simulink model "SIL_OlfatiSaber"  (R2021b)
settings: Solver=FixedStepDiscrete  StartTime=0  StopTime=T  FixedStep=0.01  RelTol=1e-3  EnableMultiTasking=on
model workspace (MAT data in the model file):
  SL_ROS_VariableLengthArrays_MaxSizes : object (value not decoded)
values from neighbouring files (symbols this model uses):
  airspeed_ref = 42    [start_swarm.m]
  altitude_ref = 300    [start_swarm.m]
  N_Waypoints = size(Waypoints,1)    [start_swarm.m]
  radius_waypoint = 200    [start_swarm.m]
  Waypoints = [1200 -1000 ... (first row only)    [start_swarm.m]
undefined symbols (not defined in the file or in its folder): DiscIntNeverNeededParam, Elevators, p_swarm, Propeller, RightAileron, RightFlap, Rudder
libraries: robotlib x36, slpidlib x15, eeGeneralControl x5, simulink x5
(part 3 of 5)

== system SIL_OlfatiSaber/UAV 5/Low-level/Guidance Algorithm ==
  yaw : Inport
  x : Inport  Port=2
  y : Inport  Port=3
  x ref : Inport  Port=4
  y ref : Inport  Port=5
  Atan2 : Trigonometry  Operator=atan2
  Constant : Constant
  Constant1 : Constant  Value=0
  Constant2 : Constant  Value=1.2
  Constant3 : Constant  Value=10
  Discrete PID : slpidlib/PID Controller  Controller=PID  Form=Parallel  TimeDomain=Discrete-time  UseExternalTs=off  SampleTime=-1  IntegratorMethod=Forward Euler  FilterMethod=Forward Euler  ControllerParametersSource=external  P=1  I=1  D=0  UseFilter=on  N=100  TunerSelectOption=Transfer Function Based (PID Tuner App)  InitialConditionSource=internal  InitialConditionForIntegrator=0  InitialConditionForFilter=0  DifferentiatorICPrevScaledInput=0  ExternalReset=none  TrackingMode=off  Kt=1  LimitOutput=off  SatLimitsSource=internal  UpperSaturationLimit=inf  LowerSaturationLimit=-inf  LinearizeAsGain=on  AntiWindupMode=none  Kb=1  POutMin=[]  POutMax=[]  IOutMin=[]  IOutMax=[]  DOutMin=[]  DOutMax=[]  NOutMin=[]  NOutMax=[]  SumOutMin=[]  SumOutMax=[]  SaturationOutMin=[]  SaturationOutMax=[]  PParamMin=[]  PParamMax=[]  IParamMin=[]  IParamMax=[]  DParamMin=[]  DParamMax=[]  NParamMin=[]  NParamMax=[]  KbParamMin=[]  KbParamMax=[]  KtParamMin=[]  KtParamMax=[]  KbOutMin=[]  KbOutMax=[]  KtOutMin=[]  KtOutMax=[]  IntegratorOutMin=[]  IntegratorOutMax=[]  FilterOutMin=[]  FilterOutMax=[]  SumI1OutMin=[]  SumI1OutMax=[]  SumI2OutMin=[]  SumI2OutMax=[]  SumI3OutMin=[]  SumI3OutMax=[]  SumI4OutMin=[]  SumI4OutMax=[]  SumDOutMin=[]  SumDOutMax=[]  DifferentiatorOutMin=[]  DifferentiatorOutMax=[]  FilterDiffOutCoefMin=[]  FilterDiffOutCoefMax=[]  ReciprocalOutMin=[]  ReciprocalOutMax=[]  SumDenOutMin=[]  SumDenOutMax=[]  SumNumOutMin=[]  SumNumOutMax=[]  DivideOutMin=[]  DivideOutMax=[]  UdiffTsProdOutMin=[]  UdiffTsProdOutMax=[]  NTsProdOutMin=[]  NTsProdOutMax=[]  UintegralTsProdOutMin=[]  UintegralTsProdOutMax=[]  UngainTsProdOutMin=[]  UngainTsProdOutMax=[]  IntegratorContinuousStateAttributes=''  IntegratorStateMustResolveToSignalObject=off  IntegratorRTWStateStorageClass=Auto  FilterContinuousStateAttributes=''  FilterStateMustResolveToSignalObject=off  FilterRTWStateStorageClass=Auto  ParallelPVariant=ExternalParameters  IdealPVariant=Disabled  IVariant=ExternalParameters  DVariant=ExternalParameters  IntegratorVariant=Discrete  SatVariant=Disabled  AWVariant=Passthrough  PCopyVariant=Disabled  TRVariant=Disabled  FdbkBlocksVariant=Forward  IdealPFdbkVariant=Disabled  SatFdbkVariant=Disabled  DerivativeFilterVariant=ForwardEulerFilter  NVariant=ExternalParameters  NCopyVariant=Disabled  FilterICVariant=InternalICsFilter  IntegratorICVariant=InternalICs  ExternalResetVariant=Disabled  TRSumVariant=Passthrough  SumFdbkVariant=Disabled  SumVariant=Sum_PID  TsampFilterVariant=InternalTs  TsampNgainVariant=Passthrough  TsampIntegralVariant=Passthrough  ExternalSaturationOutDataTypeStr=Inherit: Same as second input
  Gain : Gain  Gain=1.67
  Gain1 : Gain  Gain=-1
  Mux1 : Mux  Inputs=2
  Mux2 : Mux  Inputs=2
  Mux3 : Mux  Inputs=2
  Saturation : Saturate  UpperLimit=0.226893  LowerLimit=-0.226893
  Sum2 : Sum  Inputs=|+-
  Sum3 : Sum  Inputs=|+-
  Sum4 : Sum  Inputs=|+-
  roll_ref : Outport
  yaw_error : Outport  Port=2
  positions : Outport  Port=3
  wires:
  Mux1/1 -> Mux3/1
  Mux2/1 -> Mux3/2
  Saturation/1 -> Gain1/1
  Sum3/1 -> Atan2/1
  y/1 -> Sum3/2, Mux2/2
  y ref/1 -> Mux2/1, Sum3/1
  x ref/1 -> Mux1/1, Sum2/1
  x/1 -> Sum2/2, Mux1/2
  Sum2/1 -> Atan2/2
  Atan2/1 -> Sum4/1
  yaw/1 -> Sum4/2
  Mux3/1 -> positions/1
  Discrete PID/1 -> Saturation/1
  Sum4/1 -> yaw_error/1, Gain/1
  Gain1/1 -> roll_ref/1
  Constant/1 -> Discrete PID/2
  Constant1/1 -> Discrete PID/3
  Constant2/1 -> Discrete PID/4
  Constant3/1 -> Discrete PID/5
  Gain/1 -> Discrete PID/1

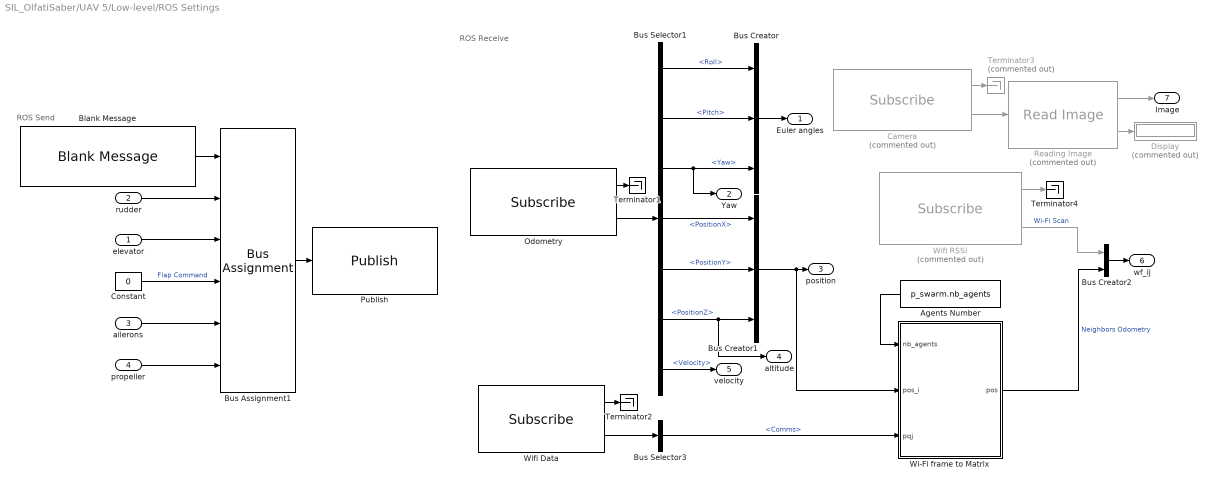
== system SIL_OlfatiSaber/UAV 5/Low-level/ROS Settings ==
  note: ROS Receive
  note: ROS Send
  elevator : Inport
  rudder : Inport  Port=2
  ailerons : Inport  Port=3
  propeller : Inport  Port=4
  Agents Number : Constant  Value=p_swarm.nb_agents
  Blank Message : robotlib/Blank Message  messageClass=Message  entityType=cosmus_messages/Control_Surfaces  messageType=cosmus_messages/Control_Surfaces  SampleTime=-1  legacyBusStruct=off
  Bus Assignment1 : BusAssignment  AssignedSignals=Rudder,Elevators,RightFlap,RightAileron,Propeller
  Bus Creator : BusCreator  Inputs=3
  Bus Creator1 : BusCreator  Inputs=3
  Bus Creator2 : BusCreator  Inputs=2
  Bus Selector1 : BusSelector  OutputSignals=Roll,Pitch,Yaw,PositionX,PositionY,PositionZ,Velocity
  Bus Selector3 : BusSelector  OutputSignals=Comms
  Camera : robotlib/Subscribe  Commented=on  topicSource=Select from ROS network  topic=/uav1/camera/image_raw  messageType=sensor_msgs/Image  SampleTime=-1  legacyBusStruct=off  messageQueueLength=1
  Constant : Constant  Value=0
  Display : Display  Commented=on
  Odometry : robotlib/Subscribe  topicSource=Select from ROS network  topic=/uav5/ground_truth/Odometry  messageType=cosmus_communication/Odom  SampleTime=-1  legacyBusStruct=off  messageQueueLength=1
  Publish : robotlib/Publish  topicSource=Select from ROS network  topic=/uav5/command  messageType=cosmus_messages/Control_Surfaces  legacyBusStruct=off  messageQueueLength=1
  Reading Image : robotlib/Read Image  Commented=on  MaximumImageSize=[240, 360]  ImageEncoding=rgb8  ShowAlphaOutput=off  ShowErrorCodeOutput=on  VariableSizeOutputs=off
      settings: SourceProductBaseCode=RR
  Terminator1 : Terminator
  Terminator2 : Terminator
  Terminator3 : Terminator  Commented=on
  Terminator4 : Terminator
  Wi-Fi frame to Matrix : MATLAB Function  TreatAsAtomicUnit=on
  Wifi Data : robotlib/Subscribe  topicSource=Select from ROS network  topic=/uav5/wifi_receiver/data  messageType=cosmus_messages/NetworkComm  SampleTime=-1  legacyBusStruct=off  messageQueueLength=1
  Wifi RSSI : robotlib/Subscribe  Commented=on  topicSource=Select from ROS network  topic=/uav1/wifi_receiver/wifi_scan  messageType=cosmus_messages/WifiSignals  SampleTime=-1  legacyBusStruct=off  messageQueueLength=1
  Euler angles : Outport
  Yaw : Outport  Port=2
  position : Outport  Port=3
  altitude : Outport  Port=4
  velocity : Outport  Port=5
  wf_ij : Outport  Port=6
  Image : Outport  Port=7
  wires:
  Odometry/1 -> Terminator1/1
  Blank Message/1 -> Bus Assignment1/1
  Bus Selector1/3 -> Bus Creator/3, Yaw/1  "<Yaw>"
  Bus Creator/1 -> Euler angles/1
  Bus Selector1/1 -> Bus Creator/1  "<Roll>"
  Bus Selector1/2 -> Bus Creator/2  "<Pitch>"
  Constant/1 -> Bus Assignment1/4  "Flap Command"
  Bus Assignment1/1 -> Publish/1
  Odometry/2 -> Bus Selector1/1
  Bus Selector1/4 -> Bus Creator1/1  "<PositionX>"
  Bus Selector1/5 -> Bus Creator1/2  "<PositionY>"
  Bus Selector1/6 -> Bus Creator1/3, altitude/1  "<PositionZ>"
  propeller/1 -> Bus Assignment1/6
  ailerons/1 -> Bus Assignment1/5
  elevator/1 -> Bus Assignment1/3
  Bus Selector1/7 -> velocity/1  "<Velocity>"
  rudder/1 -> Bus Assignment1/2
  Wifi Data/1 -> Terminator2/1
  Wifi Data/2 -> Bus Selector3/1
  Bus Selector3/1 -> Wi-Fi frame to Matrix/3(pqj)  "<Comms>"
  Agents Number/1 -> Wi-Fi frame to Matrix/1(nb_agents)
  Bus Creator1/1 -> position/1, Wi-Fi frame to Matrix/2(pos_i)
  Wi-Fi frame to Matrix/1(pos) -> Bus Creator2/2  "Neighbors Odometry"
  Camera/2 -> Reading Image/1
  Reading Image/1 -> Image/1
  Reading Image/2 -> Display/1
  Camera/1 -> Terminator3/1
  Wifi RSSI/1 -> Terminator4/1
  Wifi RSSI/2 -> Bus Creator2/1  "Wi-Fi Scan"
  Bus Creator2/1 -> wf_ij/1

== system SIL_OlfatiSaber/UAV 5/Low-level/Vision ==
  Image : Inport
  Video Viewer : VideoViewer  Commented=on  FigPos=[505 744 418 304]
  wires:
  Image/1 -> Video Viewer/1

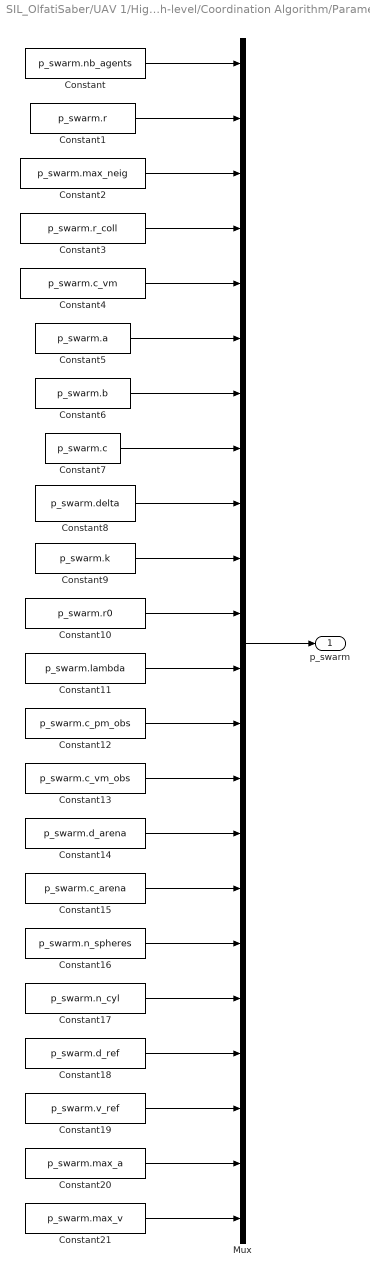
== system SIL_OlfatiSaber/UAV 1/High-level/Coordination Algorithm/Parameters ==
  Constant : Constant  Value=p_swarm.nb_agents
  Constant1 : Constant  Value=p_swarm.r
  Constant10 : Constant  Value=p_swarm.r0
  Constant11 : Constant  Value=p_swarm.lambda
  Constant12 : Constant  Value=p_swarm.c_pm_obs
  Constant13 : Constant  Value=p_swarm.c_vm_obs
  Constant14 : Constant  Value=p_swarm.d_arena
  Constant15 : Constant  Value=p_swarm.c_arena
  Constant16 : Constant  Value=p_swarm.n_spheres
  Constant17 : Constant  Value=p_swarm.n_cyl
  Constant18 : Constant  Value=p_swarm.d_ref
  Constant19 : Constant  Value=p_swarm.v_ref
  Constant2 : Constant  Value=p_swarm.max_neig
  Constant20 : Constant  Value=p_swarm.max_a
  Constant21 : Constant  Value=p_swarm.max_v
  Constant3 : Constant  Value=p_swarm.r_coll
  Constant4 : Constant  Value=p_swarm.c_vm
  Constant5 : Constant  Value=p_swarm.a
  Constant6 : Constant  Value=p_swarm.b
  Constant7 : Constant  Value=p_swarm.c
  Constant8 : Constant  Value=p_swarm.delta
  Constant9 : Constant  Value=p_swarm.k
  Mux : Mux  Inputs=22
  p_swarm : Outport
  wires:
  Mux/1 -> p_swarm/1
  Constant21/1 -> Mux/22
  Constant20/1 -> Mux/21
  Constant19/1 -> Mux/20
  Constant18/1 -> Mux/19
  Constant17/1 -> Mux/18
  Constant16/1 -> Mux/17
  Constant15/1 -> Mux/16
  Constant14/1 -> Mux/15
  Constant13/1 -> Mux/14
  Constant12/1 -> Mux/13
  Constant11/1 -> Mux/12
  Constant10/1 -> Mux/11
  Constant9/1 -> Mux/10
  Constant8/1 -> Mux/9
  Constant7/1 -> Mux/8
  Constant6/1 -> Mux/7
  Constant5/1 -> Mux/6
  Constant4/1 -> Mux/5
  Constant3/1 -> Mux/4
  Constant2/1 -> Mux/3
  Constant1/1 -> Mux/2
  Constant/1 -> Mux/1

== system SIL_OlfatiSaber/UAV 1/Low-level/Autopilot/Altitude Control ==
  Altitude Ref : Inport
  Altitude : Inport  Port=2
  Constant : Constant
  Constant1 : Constant  Value=0.00
  Constant2 : Constant  Value=0.0162
  Constant3 : Constant  Value=10
  Discrete PID : slpidlib/PID Controller  Controller=PID  Form=Parallel  TimeDomain=Discrete-time  UseExternalTs=off  SampleTime=-1  IntegratorMethod=Forward Euler  FilterMethod=Forward Euler  ControllerParametersSource=external  P=1  I=1  D=0  UseFilter=on  N=100  TunerSelectOption=Transfer Function Based (PID Tuner App)  InitialConditionSource=internal  InitialConditionForIntegrator=0  InitialConditionForFilter=0  DifferentiatorICPrevScaledInput=0  ExternalReset=none  TrackingMode=off  Kt=1  LimitOutput=off  SatLimitsSource=internal  UpperSaturationLimit=inf  LowerSaturationLimit=-inf  LinearizeAsGain=on  AntiWindupMode=none  Kb=1  POutMin=[]  POutMax=[]  IOutMin=[]  IOutMax=[]  DOutMin=[]  DOutMax=[]  NOutMin=[]  NOutMax=[]  SumOutMin=[]  SumOutMax=[]  SaturationOutMin=[]  SaturationOutMax=[]  PParamMin=[]  PParamMax=[]  IParamMin=[]  IParamMax=[]  DParamMin=[]  DParamMax=[]  NParamMin=[]  NParamMax=[]  KbParamMin=[]  KbParamMax=[]  KtParamMin=[]  KtParamMax=[]  KbOutMin=[]  KbOutMax=[]  KtOutMin=[]  KtOutMax=[]  IntegratorOutMin=[]  IntegratorOutMax=[]  FilterOutMin=[]  FilterOutMax=[]  SumI1OutMin=[]  SumI1OutMax=[]  SumI2OutMin=[]  SumI2OutMax=[]  SumI3OutMin=[]  SumI3OutMax=[]  SumI4OutMin=[]  SumI4OutMax=[]  SumDOutMin=[]  SumDOutMax=[]  DifferentiatorOutMin=[]  DifferentiatorOutMax=[]  FilterDiffOutCoefMin=[]  FilterDiffOutCoefMax=[]  ReciprocalOutMin=[]  ReciprocalOutMax=[]  SumDenOutMin=[]  SumDenOutMax=[]  SumNumOutMin=[]  SumNumOutMax=[]  DivideOutMin=[]  DivideOutMax=[]  UdiffTsProdOutMin=[]  UdiffTsProdOutMax=[]  NTsProdOutMin=[]  NTsProdOutMax=[]  UintegralTsProdOutMin=[]  UintegralTsProdOutMax=[]  UngainTsProdOutMin=[]  UngainTsProdOutMax=[]  IntegratorContinuousStateAttributes=''  IntegratorStateMustResolveToSignalObject=off  IntegratorRTWStateStorageClass=Auto  FilterContinuousStateAttributes=''  FilterStateMustResolveToSignalObject=off  FilterRTWStateStorageClass=Auto  ParallelPVariant=ExternalParameters  IdealPVariant=Disabled  IVariant=ExternalParameters  DVariant=ExternalParameters  IntegratorVariant=Discrete  SatVariant=Disabled  AWVariant=Passthrough  PCopyVariant=Disabled  TRVariant=Disabled  FdbkBlocksVariant=Forward  IdealPFdbkVariant=Disabled  SatFdbkVariant=Disabled  DerivativeFilterVariant=ForwardEulerFilter  NVariant=ExternalParameters  NCopyVariant=Disabled  FilterICVariant=InternalICsFilter  IntegratorICVariant=InternalICs  ExternalResetVariant=Disabled  TRSumVariant=Passthrough  SumFdbkVariant=Disabled  SumVariant=Sum_PID  TsampFilterVariant=InternalTs  TsampNgainVariant=Passthrough  TsampIntegralVariant=Passthrough  ExternalSaturationOutDataTypeStr=Inherit: Same as second input
  Gain : Gain  Gain=0.1
  Saturation : Saturate  UpperLimit=0.78  LowerLimit=-0.78
  Sum : Sum  Inputs=|+-
  Pitch_ref : Outport
  altitude_error : Outport  Port=2
  wires:
  Saturation/1 -> Pitch_ref/1
  Altitude Ref/1 -> Sum/1
  Altitude/1 -> Sum/2
  Sum/1 -> altitude_error/1, Gain/1
  Constant/1 -> Discrete PID/2
  Constant1/1 -> Discrete PID/3
  Constant2/1 -> Discrete PID/4
  Constant3/1 -> Discrete PID/5
  Discrete PID/1 -> Saturation/1
  Gain/1 -> Discrete PID/1

== system SIL_OlfatiSaber/UAV 1/Low-level/Autopilot/Attitude Control ==
  Pitch Ref : Inport
  Roll_ref : Inport  Port=2
  Euler angles : Inport  Port=3
  Bus Selector1 : BusSelector  OutputSignals=Pitch,Yaw,Roll
  Sum1 : Sum  Inputs=|+-
  Sum3 : Sum  Inputs=+-|
  Terminator : Terminator
  pitch_error : Outport
  roll_error : Outport  Port=2
  wires:
  Euler angles/1 -> Bus Selector1/1
  Sum1/1 -> roll_error/1
  Sum3/1 -> pitch_error/1
  Roll_ref/1 -> Sum1/1
  Bus Selector1/1 -> Sum3/2  "<Pitch>"
  Pitch Ref/1 -> Sum3/1
  Bus Selector1/3 -> Sum1/2  "<Roll>"
  Bus Selector1/2 -> Terminator/1  "<Yaw>"

== system SIL_OlfatiSaber/UAV 1/Low-level/Autopilot/Takeoff ==
  Elevator Command : Inport
  Ailerons Command : Inport  Port=2
  Propeller Command : Inport  Port=3
  Altitude : Inport  Port=4
  Constant1 : Constant  Value=0.0436332
  Constant2 : Constant  Value=0.017
  Constant3 : Constant  Value=0.8
  Constant4 : Constant  Value=0
  Constant5 : Constant  Value=-0.035
  GreaterThanOrEqual : RelationalOperator  OutDataTypeStr=boolean  RndMeth=Simplest
  Switch{1..4} (4 alike) : Switch  Criteria=u2 ~= 0
  altitude takeoff : Constant  Value=5
  profundor : Outport
  aileron : Outport  Port=2
  throtlle : Outport  Port=3
  rudder : Outport  Port=4
  wires:
  Elevator Command/1 -> Switch3/1
  Switch3/1 -> profundor/1
  Ailerons Command/1 -> Switch1/1
  Switch1/1 -> aileron/1
  Switch2/1 -> throtlle/1
  Propeller Command/1 -> Switch2/1
  Constant1/1 -> Switch3/3
  Constant2/1 -> Switch1/3
  Constant3/1 -> Switch2/3
  altitude takeoff/1 -> GreaterThanOrEqual/2
  Altitude/1 -> GreaterThanOrEqual/1
  GreaterThanOrEqual/1 -> Switch4/2, Switch3/2, Switch1/2, Switch2/2
  Constant4/1 -> Switch4/1
  Constant5/1 -> Switch4/3
  Switch4/1 -> rudder/1

== system SIL_OlfatiSaber/UAV 1/Low-level/Autopilot/Velocity Control ==
  Velocity Ref : Inport
  Velocity : Inport  Port=2
  Constant : Constant
  Constant1 : Constant  Value=0.00
  Constant2 : Constant  Value=0.009
  Constant3 : Constant  Value=10
  Discrete PID : slpidlib/PID Controller  Controller=PID  Form=Parallel  TimeDomain=Discrete-time  UseExternalTs=off  SampleTime=-1  IntegratorMethod=Forward Euler  FilterMethod=Forward Euler  ControllerParametersSource=external  P=1  I=1  D=0  UseFilter=on  N=100  TunerSelectOption=Transfer Function Based (PID Tuner App)  InitialConditionSource=internal  InitialConditionForIntegrator=0  InitialConditionForFilter=0  DifferentiatorICPrevScaledInput=0  ExternalReset=none  TrackingMode=off  Kt=1  LimitOutput=off  SatLimitsSource=internal  UpperSaturationLimit=inf  LowerSaturationLimit=-inf  LinearizeAsGain=on  AntiWindupMode=none  Kb=1  POutMin=[]  POutMax=[]  IOutMin=[]  IOutMax=[]  DOutMin=[]  DOutMax=[]  NOutMin=[]  NOutMax=[]  SumOutMin=[]  SumOutMax=[]  SaturationOutMin=[]  SaturationOutMax=[]  PParamMin=[]  PParamMax=[]  IParamMin=[]  IParamMax=[]  DParamMin=[]  DParamMax=[]  NParamMin=[]  NParamMax=[]  KbParamMin=[]  KbParamMax=[]  KtParamMin=[]  KtParamMax=[]  KbOutMin=[]  KbOutMax=[]  KtOutMin=[]  KtOutMax=[]  IntegratorOutMin=[]  IntegratorOutMax=[]  FilterOutMin=[]  FilterOutMax=[]  SumI1OutMin=[]  SumI1OutMax=[]  SumI2OutMin=[]  SumI2OutMax=[]  SumI3OutMin=[]  SumI3OutMax=[]  SumI4OutMin=[]  SumI4OutMax=[]  SumDOutMin=[]  SumDOutMax=[]  DifferentiatorOutMin=[]  DifferentiatorOutMax=[]  FilterDiffOutCoefMin=[]  FilterDiffOutCoefMax=[]  ReciprocalOutMin=[]  ReciprocalOutMax=[]  SumDenOutMin=[]  SumDenOutMax=[]  SumNumOutMin=[]  SumNumOutMax=[]  DivideOutMin=[]  DivideOutMax=[]  UdiffTsProdOutMin=[]  UdiffTsProdOutMax=[]  NTsProdOutMin=[]  NTsProdOutMax=[]  UintegralTsProdOutMin=[]  UintegralTsProdOutMax=[]  UngainTsProdOutMin=[]  UngainTsProdOutMax=[]  IntegratorContinuousStateAttributes=''  IntegratorStateMustResolveToSignalObject=off  IntegratorRTWStateStorageClass=Auto  FilterContinuousStateAttributes=''  FilterStateMustResolveToSignalObject=off  FilterRTWStateStorageClass=Auto  ParallelPVariant=ExternalParameters  IdealPVariant=Disabled  IVariant=ExternalParameters  DVariant=ExternalParameters  IntegratorVariant=Discrete  SatVariant=Disabled  AWVariant=Passthrough  PCopyVariant=Disabled  TRVariant=Disabled  FdbkBlocksVariant=Forward  IdealPFdbkVariant=Disabled  SatFdbkVariant=Disabled  DerivativeFilterVariant=ForwardEulerFilter  NVariant=ExternalParameters  NCopyVariant=Disabled  FilterICVariant=InternalICsFilter  IntegratorICVariant=InternalICs  ExternalResetVariant=Disabled  TRSumVariant=Passthrough  SumFdbkVariant=Disabled  SumVariant=Sum_PID  TsampFilterVariant=InternalTs  TsampNgainVariant=Passthrough  TsampIntegralVariant=Passthrough  ExternalSaturationOutDataTypeStr=Inherit: Same as second input
  K_prop : Gain  Gain=0.1
  Sum1 : Sum  Inputs=|++
  Sum7 : Sum  Inputs=|+-
  propeller_ref : Constant  Value=0.64
  propeller_cmd : Outport
  velocity_error : Outport  Port=2
  wires:
  Velocity/1 -> Sum7/2
  Velocity Ref/1 -> Sum7/1
  Sum7/1 -> velocity_error/1, K_prop/1
  Sum1/1 -> propeller_cmd/1
  propeller_ref/1 -> Sum1/2
  Constant3/1 -> Discrete PID/5
  Constant/1 -> Discrete PID/2
  Discrete PID/1 -> Sum1/1
  Constant1/1 -> Discrete PID/3
  K_prop/1 -> Discrete PID/1
  Constant2/1 -> Discrete PID/4

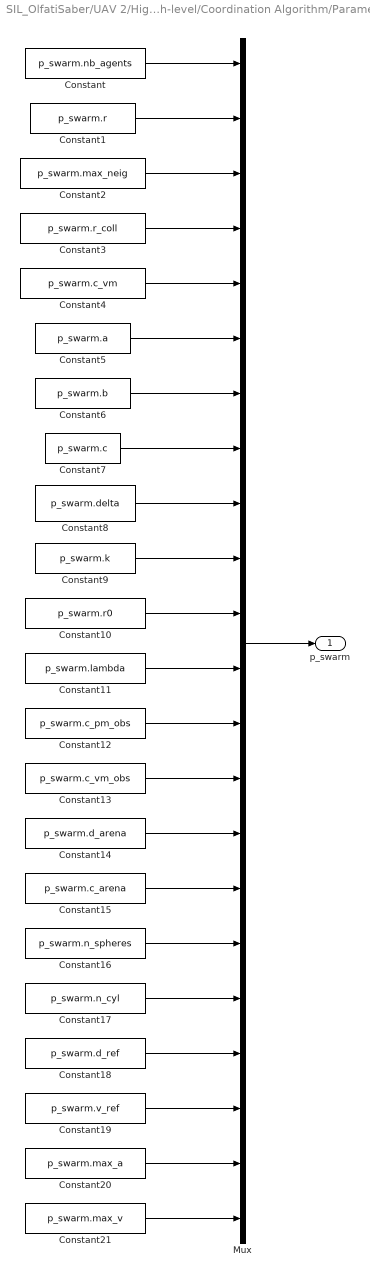
== system SIL_OlfatiSaber/UAV 2/High-level/Coordination Algorithm/Parameters ==
  Constant : Constant  Value=p_swarm.nb_agents
  Constant1 : Constant  Value=p_swarm.r
  Constant10 : Constant  Value=p_swarm.r0
  Constant11 : Constant  Value=p_swarm.lambda
  Constant12 : Constant  Value=p_swarm.c_pm_obs
  Constant13 : Constant  Value=p_swarm.c_vm_obs
  Constant14 : Constant  Value=p_swarm.d_arena
  Constant15 : Constant  Value=p_swarm.c_arena
  Constant16 : Constant  Value=p_swarm.n_spheres
  Constant17 : Constant  Value=p_swarm.n_cyl
  Constant18 : Constant  Value=p_swarm.d_ref
  Constant19 : Constant  Value=p_swarm.v_ref
  Constant2 : Constant  Value=p_swarm.max_neig
  Constant20 : Constant  Value=p_swarm.max_a
  Constant21 : Constant  Value=p_swarm.max_v
  Constant3 : Constant  Value=p_swarm.r_coll
  Constant4 : Constant  Value=p_swarm.c_vm
  Constant5 : Constant  Value=p_swarm.a
  Constant6 : Constant  Value=p_swarm.b
  Constant7 : Constant  Value=p_swarm.c
  Constant8 : Constant  Value=p_swarm.delta
  Constant9 : Constant  Value=p_swarm.k
  Mux : Mux  Inputs=22
  p_swarm : Outport
  wires:
  Mux/1 -> p_swarm/1
  Constant21/1 -> Mux/22
  Constant20/1 -> Mux/21
  Constant19/1 -> Mux/20
  Constant18/1 -> Mux/19
  Constant17/1 -> Mux/18
  Constant16/1 -> Mux/17
  Constant15/1 -> Mux/16
  Constant14/1 -> Mux/15
  Constant13/1 -> Mux/14
  Constant12/1 -> Mux/13
  Constant11/1 -> Mux/12
  Constant10/1 -> Mux/11
  Constant9/1 -> Mux/10
  Constant8/1 -> Mux/9
  Constant7/1 -> Mux/8
  Constant6/1 -> Mux/7
  Constant5/1 -> Mux/6
  Constant4/1 -> Mux/5
  Constant3/1 -> Mux/4
  Constant2/1 -> Mux/3
  Constant1/1 -> Mux/2
  Constant/1 -> Mux/1

== system SIL_OlfatiSaber/UAV 2/Low-level/Autopilot/Altitude Control ==
  Altitude Ref : Inport
  Altitude : Inport  Port=2
  Constant : Constant
  Constant1 : Constant  Value=0.00
  Constant2 : Constant  Value=0.0162
  Constant3 : Constant  Value=10
  Discrete PID : slpidlib/PID Controller  Controller=PID  Form=Parallel  TimeDomain=Discrete-time  UseExternalTs=off  SampleTime=-1  IntegratorMethod=Forward Euler  FilterMethod=Forward Euler  ControllerParametersSource=external  P=1  I=1  D=0  UseFilter=on  N=100  TunerSelectOption=Transfer Function Based (PID Tuner App)  InitialConditionSource=internal  InitialConditionForIntegrator=0  InitialConditionForFilter=0  DifferentiatorICPrevScaledInput=0  ExternalReset=none  TrackingMode=off  Kt=1  LimitOutput=off  SatLimitsSource=internal  UpperSaturationLimit=inf  LowerSaturationLimit=-inf  LinearizeAsGain=on  AntiWindupMode=none  Kb=1  POutMin=[]  POutMax=[]  IOutMin=[]  IOutMax=[]  DOutMin=[]  DOutMax=[]  NOutMin=[]  NOutMax=[]  SumOutMin=[]  SumOutMax=[]  SaturationOutMin=[]  SaturationOutMax=[]  PParamMin=[]  PParamMax=[]  IParamMin=[]  IParamMax=[]  DParamMin=[]  DParamMax=[]  NParamMin=[]  NParamMax=[]  KbParamMin=[]  KbParamMax=[]  KtParamMin=[]  KtParamMax=[]  KbOutMin=[]  KbOutMax=[]  KtOutMin=[]  KtOutMax=[]  IntegratorOutMin=[]  IntegratorOutMax=[]  FilterOutMin=[]  FilterOutMax=[]  SumI1OutMin=[]  SumI1OutMax=[]  SumI2OutMin=[]  SumI2OutMax=[]  SumI3OutMin=[]  SumI3OutMax=[]  SumI4OutMin=[]  SumI4OutMax=[]  SumDOutMin=[]  SumDOutMax=[]  DifferentiatorOutMin=[]  DifferentiatorOutMax=[]  FilterDiffOutCoefMin=[]  FilterDiffOutCoefMax=[]  ReciprocalOutMin=[]  ReciprocalOutMax=[]  SumDenOutMin=[]  SumDenOutMax=[]  SumNumOutMin=[]  SumNumOutMax=[]  DivideOutMin=[]  DivideOutMax=[]  UdiffTsProdOutMin=[]  UdiffTsProdOutMax=[]  NTsProdOutMin=[]  NTsProdOutMax=[]  UintegralTsProdOutMin=[]  UintegralTsProdOutMax=[]  UngainTsProdOutMin=[]  UngainTsProdOutMax=[]  IntegratorContinuousStateAttributes=''  IntegratorStateMustResolveToSignalObject=off  IntegratorRTWStateStorageClass=Auto  FilterContinuousStateAttributes=''  FilterStateMustResolveToSignalObject=off  FilterRTWStateStorageClass=Auto  ParallelPVariant=ExternalParameters  IdealPVariant=Disabled  IVariant=ExternalParameters  DVariant=ExternalParameters  IntegratorVariant=Discrete  SatVariant=Disabled  AWVariant=Passthrough  PCopyVariant=Disabled  TRVariant=Disabled  FdbkBlocksVariant=Forward  IdealPFdbkVariant=Disabled  SatFdbkVariant=Disabled  DerivativeFilterVariant=ForwardEulerFilter  NVariant=ExternalParameters  NCopyVariant=Disabled  FilterICVariant=InternalICsFilter  IntegratorICVariant=InternalICs  ExternalResetVariant=Disabled  TRSumVariant=Passthrough  SumFdbkVariant=Disabled  SumVariant=Sum_PID  TsampFilterVariant=InternalTs  TsampNgainVariant=Passthrough  TsampIntegralVariant=Passthrough  ExternalSaturationOutDataTypeStr=Inherit: Same as second input
  Gain : Gain  Gain=0.1
  Saturation : Saturate  UpperLimit=0.78  LowerLimit=-0.78
  Sum : Sum  Inputs=|+-
  Pitch_ref : Outport
  altitude_error : Outport  Port=2
  wires:
  Saturation/1 -> Pitch_ref/1
  Altitude Ref/1 -> Sum/1
  Altitude/1 -> Sum/2
  Sum/1 -> altitude_error/1, Gain/1
  Constant/1 -> Discrete PID/2
  Constant1/1 -> Discrete PID/3
  Constant2/1 -> Discrete PID/4
  Constant3/1 -> Discrete PID/5
  Discrete PID/1 -> Saturation/1
  Gain/1 -> Discrete PID/1

== system SIL_OlfatiSaber/UAV 2/Low-level/Autopilot/Attitude Control ==
  Pitch Ref : Inport
  Roll_ref : Inport  Port=2
  Euler angles : Inport  Port=3
  Bus Selector1 : BusSelector  OutputSignals=Pitch,Yaw,Roll
  Sum1 : Sum  Inputs=|+-
  Sum3 : Sum  Inputs=+-|
  Terminator : Terminator
  pitch_error : Outport
  roll_error : Outport  Port=2
  wires:
  Euler angles/1 -> Bus Selector1/1
  Sum1/1 -> roll_error/1
  Sum3/1 -> pitch_error/1
  Roll_ref/1 -> Sum1/1
  Bus Selector1/1 -> Sum3/2  "<Pitch>"
  Pitch Ref/1 -> Sum3/1
  Bus Selector1/3 -> Sum1/2  "<Roll>"
  Bus Selector1/2 -> Terminator/1  "<Yaw>"

== system SIL_OlfatiSaber/UAV 2/Low-level/Autopilot/Takeoff ==
  Elevator Command : Inport
  Ailerons Command : Inport  Port=2
  Propeller Command : Inport  Port=3
  Altitude : Inport  Port=4
  Constant1 : Constant  Value=0.0436332
  Constant2 : Constant  Value=0.017
  Constant3 : Constant  Value=0.8
  Constant4 : Constant  Value=0
  Constant5 : Constant  Value=-0.035
  GreaterThanOrEqual : RelationalOperator  OutDataTypeStr=boolean  RndMeth=Simplest
  Switch{1..4} (4 alike) : Switch  Criteria=u2 ~= 0
  altitude takeoff : Constant  Value=5
  profundor : Outport
  aileron : Outport  Port=2
  throtlle : Outport  Port=3
  rudder : Outport  Port=4
  wires:
  Elevator Command/1 -> Switch3/1
  Switch3/1 -> profundor/1
  Ailerons Command/1 -> Switch1/1
  Switch1/1 -> aileron/1
  Switch2/1 -> throtlle/1
  Propeller Command/1 -> Switch2/1
  Constant1/1 -> Switch3/3
  Constant2/1 -> Switch1/3
  Constant3/1 -> Switch2/3
  altitude takeoff/1 -> GreaterThanOrEqual/2
  Altitude/1 -> GreaterThanOrEqual/1
  GreaterThanOrEqual/1 -> Switch4/2, Switch3/2, Switch1/2, Switch2/2
  Constant4/1 -> Switch4/1
  Constant5/1 -> Switch4/3
  Switch4/1 -> rudder/1

== system SIL_OlfatiSaber/UAV 2/Low-level/Autopilot/Velocity Control ==
  Velocity Ref : Inport
  Velocity : Inport  Port=2
  Constant : Constant
  Constant1 : Constant  Value=0.00
  Constant2 : Constant  Value=0.009
  Constant3 : Constant  Value=10
  Discrete PID : slpidlib/PID Controller  Controller=PID  Form=Parallel  TimeDomain=Discrete-time  UseExternalTs=off  SampleTime=-1  IntegratorMethod=Forward Euler  FilterMethod=Forward Euler  ControllerParametersSource=external  P=1  I=1  D=0  UseFilter=on  N=100  TunerSelectOption=Transfer Function Based (PID Tuner App)  InitialConditionSource=internal  InitialConditionForIntegrator=0  InitialConditionForFilter=0  DifferentiatorICPrevScaledInput=0  ExternalReset=none  TrackingMode=off  Kt=1  LimitOutput=off  SatLimitsSource=internal  UpperSaturationLimit=inf  LowerSaturationLimit=-inf  LinearizeAsGain=on  AntiWindupMode=none  Kb=1  POutMin=[]  POutMax=[]  IOutMin=[]  IOutMax=[]  DOutMin=[]  DOutMax=[]  NOutMin=[]  NOutMax=[]  SumOutMin=[]  SumOutMax=[]  SaturationOutMin=[]  SaturationOutMax=[]  PParamMin=[]  PParamMax=[]  IParamMin=[]  IParamMax=[]  DParamMin=[]  DParamMax=[]  NParamMin=[]  NParamMax=[]  KbParamMin=[]  KbParamMax=[]  KtParamMin=[]  KtParamMax=[]  KbOutMin=[]  KbOutMax=[]  KtOutMin=[]  KtOutMax=[]  IntegratorOutMin=[]  IntegratorOutMax=[]  FilterOutMin=[]  FilterOutMax=[]  SumI1OutMin=[]  SumI1OutMax=[]  SumI2OutMin=[]  SumI2OutMax=[]  SumI3OutMin=[]  SumI3OutMax=[]  SumI4OutMin=[]  SumI4OutMax=[]  SumDOutMin=[]  SumDOutMax=[]  DifferentiatorOutMin=[]  DifferentiatorOutMax=[]  FilterDiffOutCoefMin=[]  FilterDiffOutCoefMax=[]  ReciprocalOutMin=[]  ReciprocalOutMax=[]  SumDenOutMin=[]  SumDenOutMax=[]  SumNumOutMin=[]  SumNumOutMax=[]  DivideOutMin=[]  DivideOutMax=[]  UdiffTsProdOutMin=[]  UdiffTsProdOutMax=[]  NTsProdOutMin=[]  NTsProdOutMax=[]  UintegralTsProdOutMin=[]  UintegralTsProdOutMax=[]  UngainTsProdOutMin=[]  UngainTsProdOutMax=[]  IntegratorContinuousStateAttributes=''  IntegratorStateMustResolveToSignalObject=off  IntegratorRTWStateStorageClass=Auto  FilterContinuousStateAttributes=''  FilterStateMustResolveToSignalObject=off  FilterRTWStateStorageClass=Auto  ParallelPVariant=ExternalParameters  IdealPVariant=Disabled  IVariant=ExternalParameters  DVariant=ExternalParameters  IntegratorVariant=Discrete  SatVariant=Disabled  AWVariant=Passthrough  PCopyVariant=Disabled  TRVariant=Disabled  FdbkBlocksVariant=Forward  IdealPFdbkVariant=Disabled  SatFdbkVariant=Disabled  DerivativeFilterVariant=ForwardEulerFilter  NVariant=ExternalParameters  NCopyVariant=Disabled  FilterICVariant=InternalICsFilter  IntegratorICVariant=InternalICs  ExternalResetVariant=Disabled  TRSumVariant=Passthrough  SumFdbkVariant=Disabled  SumVariant=Sum_PID  TsampFilterVariant=InternalTs  TsampNgainVariant=Passthrough  TsampIntegralVariant=Passthrough  ExternalSaturationOutDataTypeStr=Inherit: Same as second input
  K_prop : Gain  Gain=0.1
  Sum1 : Sum  Inputs=|++
  Sum7 : Sum  Inputs=|+-
  propeller_ref : Constant  Value=0.64
  propeller_cmd : Outport
  velocity_error : Outport  Port=2
  wires:
  Velocity/1 -> Sum7/2
  Velocity Ref/1 -> Sum7/1
  Sum7/1 -> velocity_error/1, K_prop/1
  Sum1/1 -> propeller_cmd/1
  propeller_ref/1 -> Sum1/2
  Constant3/1 -> Discrete PID/5
  Constant/1 -> Discrete PID/2
  Discrete PID/1 -> Sum1/1
  Constant1/1 -> Discrete PID/3
  K_prop/1 -> Discrete PID/1
  Constant2/1 -> Discrete PID/4

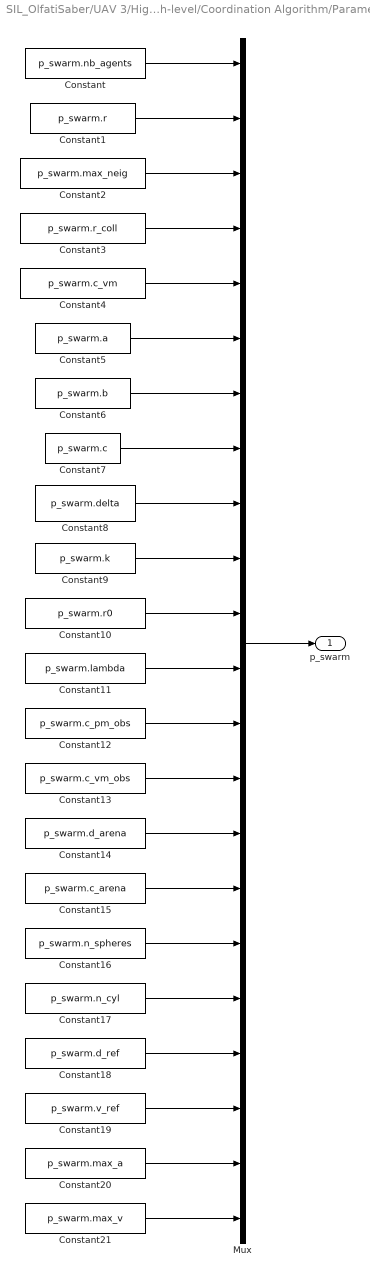
== system SIL_OlfatiSaber/UAV 3/High-level/Coordination Algorithm/Parameters ==
  Constant : Constant  Value=p_swarm.nb_agents
  Constant1 : Constant  Value=p_swarm.r
  Constant10 : Constant  Value=p_swarm.r0
  Constant11 : Constant  Value=p_swarm.lambda
  Constant12 : Constant  Value=p_swarm.c_pm_obs
  Constant13 : Constant  Value=p_swarm.c_vm_obs
  Constant14 : Constant  Value=p_swarm.d_arena
  Constant15 : Constant  Value=p_swarm.c_arena
  Constant16 : Constant  Value=p_swarm.n_spheres
  Constant17 : Constant  Value=p_swarm.n_cyl
  Constant18 : Constant  Value=p_swarm.d_ref
  Constant19 : Constant  Value=p_swarm.v_ref
  Constant2 : Constant  Value=p_swarm.max_neig
  Constant20 : Constant  Value=p_swarm.max_a
  Constant21 : Constant  Value=p_swarm.max_v
  Constant3 : Constant  Value=p_swarm.r_coll
  Constant4 : Constant  Value=p_swarm.c_vm
  Constant5 : Constant  Value=p_swarm.a
  Constant6 : Constant  Value=p_swarm.b
  Constant7 : Constant  Value=p_swarm.c
  Constant8 : Constant  Value=p_swarm.delta
  Constant9 : Constant  Value=p_swarm.k
  Mux : Mux  Inputs=22
  p_swarm : Outport
  wires:
  Mux/1 -> p_swarm/1
  Constant21/1 -> Mux/22
  Constant20/1 -> Mux/21
  Constant19/1 -> Mux/20
  Constant18/1 -> Mux/19
  Constant17/1 -> Mux/18
  Constant16/1 -> Mux/17
  Constant15/1 -> Mux/16
  Constant14/1 -> Mux/15
  Constant13/1 -> Mux/14
  Constant12/1 -> Mux/13
  Constant11/1 -> Mux/12
  Constant10/1 -> Mux/11
  Constant9/1 -> Mux/10
  Constant8/1 -> Mux/9
  Constant7/1 -> Mux/8
  Constant6/1 -> Mux/7
  Constant5/1 -> Mux/6
  Constant4/1 -> Mux/5
  Constant3/1 -> Mux/4
  Constant2/1 -> Mux/3
  Constant1/1 -> Mux/2
  Constant/1 -> Mux/1

== system SIL_OlfatiSaber/UAV 3/Low-level/Autopilot/Altitude Control ==
  Altitude Ref : Inport
  Altitude : Inport  Port=2
  Constant : Constant
  Constant1 : Constant  Value=0.00
  Constant2 : Constant  Value=0.0162
  Constant3 : Constant  Value=10
  Discrete PID : slpidlib/PID Controller  Controller=PID  Form=Parallel  TimeDomain=Discrete-time  UseExternalTs=off  SampleTime=-1  IntegratorMethod=Forward Euler  FilterMethod=Forward Euler  ControllerParametersSource=external  P=1  I=1  D=0  UseFilter=on  N=100  TunerSelectOption=Transfer Function Based (PID Tuner App)  InitialConditionSource=internal  InitialConditionForIntegrator=0  InitialConditionForFilter=0  DifferentiatorICPrevScaledInput=0  ExternalReset=none  TrackingMode=off  Kt=1  LimitOutput=off  SatLimitsSource=internal  UpperSaturationLimit=inf  LowerSaturationLimit=-inf  LinearizeAsGain=on  AntiWindupMode=none  Kb=1  POutMin=[]  POutMax=[]  IOutMin=[]  IOutMax=[]  DOutMin=[]  DOutMax=[]  NOutMin=[]  NOutMax=[]  SumOutMin=[]  SumOutMax=[]  SaturationOutMin=[]  SaturationOutMax=[]  PParamMin=[]  PParamMax=[]  IParamMin=[]  IParamMax=[]  DParamMin=[]  DParamMax=[]  NParamMin=[]  NParamMax=[]  KbParamMin=[]  KbParamMax=[]  KtParamMin=[]  KtParamMax=[]  KbOutMin=[]  KbOutMax=[]  KtOutMin=[]  KtOutMax=[]  IntegratorOutMin=[]  IntegratorOutMax=[]  FilterOutMin=[]  FilterOutMax=[]  SumI1OutMin=[]  SumI1OutMax=[]  SumI2OutMin=[]  SumI2OutMax=[]  SumI3OutMin=[]  SumI3OutMax=[]  SumI4OutMin=[]  SumI4OutMax=[]  SumDOutMin=[]  SumDOutMax=[]  DifferentiatorOutMin=[]  DifferentiatorOutMax=[]  FilterDiffOutCoefMin=[]  FilterDiffOutCoefMax=[]  ReciprocalOutMin=[]  ReciprocalOutMax=[]  SumDenOutMin=[]  SumDenOutMax=[]  SumNumOutMin=[]  SumNumOutMax=[]  DivideOutMin=[]  DivideOutMax=[]  UdiffTsProdOutMin=[]  UdiffTsProdOutMax=[]  NTsProdOutMin=[]  NTsProdOutMax=[]  UintegralTsProdOutMin=[]  UintegralTsProdOutMax=[]  UngainTsProdOutMin=[]  UngainTsProdOutMax=[]  IntegratorContinuousStateAttributes=''  IntegratorStateMustResolveToSignalObject=off  IntegratorRTWStateStorageClass=Auto  FilterContinuousStateAttributes=''  FilterStateMustResolveToSignalObject=off  FilterRTWStateStorageClass=Auto  ParallelPVariant=ExternalParameters  IdealPVariant=Disabled  IVariant=ExternalParameters  DVariant=ExternalParameters  IntegratorVariant=Discrete  SatVariant=Disabled  AWVariant=Passthrough  PCopyVariant=Disabled  TRVariant=Disabled  FdbkBlocksVariant=Forward  IdealPFdbkVariant=Disabled  SatFdbkVariant=Disabled  DerivativeFilterVariant=ForwardEulerFilter  NVariant=ExternalParameters  NCopyVariant=Disabled  FilterICVariant=InternalICsFilter  IntegratorICVariant=InternalICs  ExternalResetVariant=Disabled  TRSumVariant=Passthrough  SumFdbkVariant=Disabled  SumVariant=Sum_PID  TsampFilterVariant=InternalTs  TsampNgainVariant=Passthrough  TsampIntegralVariant=Passthrough  ExternalSaturationOutDataTypeStr=Inherit: Same as second input
  Gain : Gain  Gain=0.1
  Saturation : Saturate  UpperLimit=0.78  LowerLimit=-0.78
  Sum : Sum  Inputs=|+-
  Pitch_ref : Outport
  altitude_error : Outport  Port=2
  wires:
  Saturation/1 -> Pitch_ref/1
  Altitude Ref/1 -> Sum/1
  Altitude/1 -> Sum/2
  Sum/1 -> altitude_error/1, Gain/1
  Constant/1 -> Discrete PID/2
  Constant1/1 -> Discrete PID/3
  Constant2/1 -> Discrete PID/4
  Constant3/1 -> Discrete PID/5
  Discrete PID/1 -> Saturation/1
  Gain/1 -> Discrete PID/1

== system SIL_OlfatiSaber/UAV 3/Low-level/Autopilot/Attitude Control ==
  Pitch Ref : Inport
  Roll_ref : Inport  Port=2
  Euler angles : Inport  Port=3
  Bus Selector1 : BusSelector  OutputSignals=Pitch,Yaw,Roll
  Sum1 : Sum  Inputs=|+-
  Sum3 : Sum  Inputs=+-|
  Terminator : Terminator
  pitch_error : Outport
  roll_error : Outport  Port=2
  wires:
  Euler angles/1 -> Bus Selector1/1
  Sum1/1 -> roll_error/1
  Sum3/1 -> pitch_error/1
  Roll_ref/1 -> Sum1/1
  Bus Selector1/1 -> Sum3/2  "<Pitch>"
  Pitch Ref/1 -> Sum3/1
  Bus Selector1/3 -> Sum1/2  "<Roll>"
  Bus Selector1/2 -> Terminator/1  "<Yaw>"

== system SIL_OlfatiSaber/UAV 3/Low-level/Autopilot/Takeoff ==
  Elevator Command : Inport
  Ailerons Command : Inport  Port=2
  Propeller Command : Inport  Port=3
  Altitude : Inport  Port=4
  Constant1 : Constant  Value=0.0436332
  Constant2 : Constant  Value=0.017
  Constant3 : Constant  Value=0.8
  Constant4 : Constant  Value=0
  Constant5 : Constant  Value=-0.035
  GreaterThanOrEqual : RelationalOperator  OutDataTypeStr=boolean  RndMeth=Simplest
  Switch{1..4} (4 alike) : Switch  Criteria=u2 ~= 0
  altitude takeoff : Constant  Value=5
  profundor : Outport
  aileron : Outport  Port=2
  throtlle : Outport  Port=3
  rudder : Outport  Port=4
  wires:
  Elevator Command/1 -> Switch3/1
  Switch3/1 -> profundor/1
  Ailerons Command/1 -> Switch1/1
  Switch1/1 -> aileron/1
  Switch2/1 -> throtlle/1
  Propeller Command/1 -> Switch2/1
  Constant1/1 -> Switch3/3
  Constant2/1 -> Switch1/3
  Constant3/1 -> Switch2/3
  altitude takeoff/1 -> GreaterThanOrEqual/2
  Altitude/1 -> GreaterThanOrEqual/1
  GreaterThanOrEqual/1 -> Switch4/2, Switch3/2, Switch1/2, Switch2/2
  Constant4/1 -> Switch4/1
  Constant5/1 -> Switch4/3
  Switch4/1 -> rudder/1

== system SIL_OlfatiSaber/UAV 3/Low-level/Autopilot/Velocity Control ==
  Velocity Ref : Inport
  Velocity : Inport  Port=2
  Constant : Constant
  Constant1 : Constant  Value=0.00
  Constant2 : Constant  Value=0.009
  Constant3 : Constant  Value=10
  Discrete PID : slpidlib/PID Controller  Controller=PID  Form=Parallel  TimeDomain=Discrete-time  UseExternalTs=off  SampleTime=-1  IntegratorMethod=Forward Euler  FilterMethod=Forward Euler  ControllerParametersSource=external  P=1  I=1  D=0  UseFilter=on  N=100  TunerSelectOption=Transfer Function Based (PID Tuner App)  InitialConditionSource=internal  InitialConditionForIntegrator=0  InitialConditionForFilter=0  DifferentiatorICPrevScaledInput=0  ExternalReset=none  TrackingMode=off  Kt=1  LimitOutput=off  SatLimitsSource=internal  UpperSaturationLimit=inf  LowerSaturationLimit=-inf  LinearizeAsGain=on  AntiWindupMode=none  Kb=1  POutMin=[]  POutMax=[]  IOutMin=[]  IOutMax=[]  DOutMin=[]  DOutMax=[]  NOutMin=[]  NOutMax=[]  SumOutMin=[]  SumOutMax=[]  SaturationOutMin=[]  SaturationOutMax=[]  PParamMin=[]  PParamMax=[]  IParamMin=[]  IParamMax=[]  DParamMin=[]  DParamMax=[]  NParamMin=[]  NParamMax=[]  KbParamMin=[]  KbParamMax=[]  KtParamMin=[]  KtParamMax=[]  KbOutMin=[]  KbOutMax=[]  KtOutMin=[]  KtOutMax=[]  IntegratorOutMin=[]  IntegratorOutMax=[]  FilterOutMin=[]  FilterOutMax=[]  SumI1OutMin=[]  SumI1OutMax=[]  SumI2OutMin=[]  SumI2OutMax=[]  SumI3OutMin=[]  SumI3OutMax=[]  SumI4OutMin=[]  SumI4OutMax=[]  SumDOutMin=[]  SumDOutMax=[]  DifferentiatorOutMin=[]  DifferentiatorOutMax=[]  FilterDiffOutCoefMin=[]  FilterDiffOutCoefMax=[]  ReciprocalOutMin=[]  ReciprocalOutMax=[]  SumDenOutMin=[]  SumDenOutMax=[]  SumNumOutMin=[]  SumNumOutMax=[]  DivideOutMin=[]  DivideOutMax=[]  UdiffTsProdOutMin=[]  UdiffTsProdOutMax=[]  NTsProdOutMin=[]  NTsProdOutMax=[]  UintegralTsProdOutMin=[]  UintegralTsProdOutMax=[]  UngainTsProdOutMin=[]  UngainTsProdOutMax=[]  IntegratorContinuousStateAttributes=''  IntegratorStateMustResolveToSignalObject=off  IntegratorRTWStateStorageClass=Auto  FilterContinuousStateAttributes=''  FilterStateMustResolveToSignalObject=off  FilterRTWStateStorageClass=Auto  ParallelPVariant=ExternalParameters  IdealPVariant=Disabled  IVariant=ExternalParameters  DVariant=ExternalParameters  IntegratorVariant=Discrete  SatVariant=Disabled  AWVariant=Passthrough  PCopyVariant=Disabled  TRVariant=Disabled  FdbkBlocksVariant=Forward  IdealPFdbkVariant=Disabled  SatFdbkVariant=Disabled  DerivativeFilterVariant=ForwardEulerFilter  NVariant=ExternalParameters  NCopyVariant=Disabled  FilterICVariant=InternalICsFilter  IntegratorICVariant=InternalICs  ExternalResetVariant=Disabled  TRSumVariant=Passthrough  SumFdbkVariant=Disabled  SumVariant=Sum_PID  TsampFilterVariant=InternalTs  TsampNgainVariant=Passthrough  TsampIntegralVariant=Passthrough  ExternalSaturationOutDataTypeStr=Inherit: Same as second input
  K_prop : Gain  Gain=0.1
  Sum1 : Sum  Inputs=|++
  Sum7 : Sum  Inputs=|+-
  propeller_ref : Constant  Value=0.64
  propeller_cmd : Outport
  velocity_error : Outport  Port=2
  wires:
  Velocity/1 -> Sum7/2
  Velocity Ref/1 -> Sum7/1
  Sum7/1 -> velocity_error/1, K_prop/1
  Sum1/1 -> propeller_cmd/1
  propeller_ref/1 -> Sum1/2
  Constant3/1 -> Discrete PID/5
  Constant/1 -> Discrete PID/2
  Discrete PID/1 -> Sum1/1
  Constant1/1 -> Discrete PID/3
  K_prop/1 -> Discrete PID/1
  Constant2/1 -> Discrete PID/4

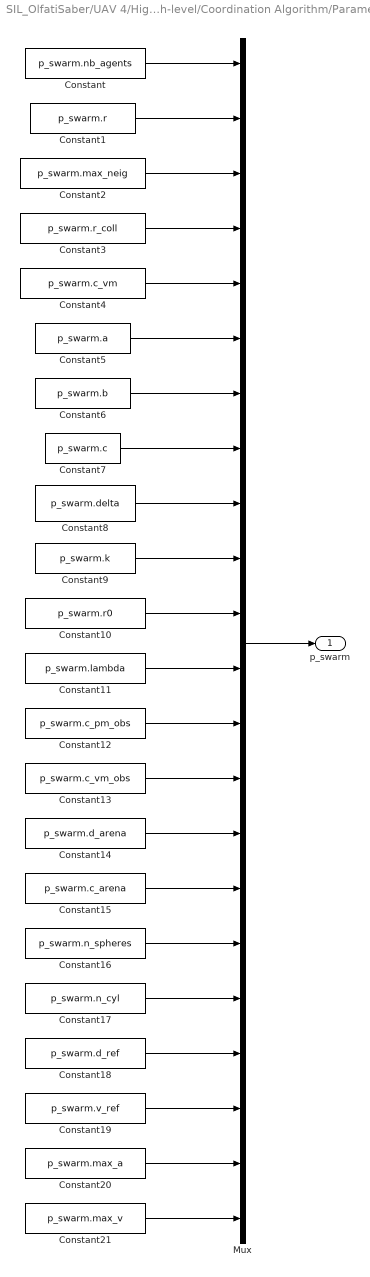
== system SIL_OlfatiSaber/UAV 4/High-level/Coordination Algorithm/Parameters ==
  Constant : Constant  Value=p_swarm.nb_agents
  Constant1 : Constant  Value=p_swarm.r
  Constant10 : Constant  Value=p_swarm.r0
  Constant11 : Constant  Value=p_swarm.lambda
  Constant12 : Constant  Value=p_swarm.c_pm_obs
  Constant13 : Constant  Value=p_swarm.c_vm_obs
  Constant14 : Constant  Value=p_swarm.d_arena
  Constant15 : Constant  Value=p_swarm.c_arena
  Constant16 : Constant  Value=p_swarm.n_spheres
  Constant17 : Constant  Value=p_swarm.n_cyl
  Constant18 : Constant  Value=p_swarm.d_ref
  Constant19 : Constant  Value=p_swarm.v_ref
  Constant2 : Constant  Value=p_swarm.max_neig
  Constant20 : Constant  Value=p_swarm.max_a
  Constant21 : Constant  Value=p_swarm.max_v
  Constant3 : Constant  Value=p_swarm.r_coll
  Constant4 : Constant  Value=p_swarm.c_vm
  Constant5 : Constant  Value=p_swarm.a
  Constant6 : Constant  Value=p_swarm.b
  Constant7 : Constant  Value=p_swarm.c
  Constant8 : Constant  Value=p_swarm.delta
  Constant9 : Constant  Value=p_swarm.k
  Mux : Mux  Inputs=22
  p_swarm : Outport
  wires:
  Mux/1 -> p_swarm/1
  Constant21/1 -> Mux/22
  Constant20/1 -> Mux/21
  Constant19/1 -> Mux/20
  Constant18/1 -> Mux/19
  Constant17/1 -> Mux/18
  Constant16/1 -> Mux/17
  Constant15/1 -> Mux/16
  Constant14/1 -> Mux/15
  Constant13/1 -> Mux/14
  Constant12/1 -> Mux/13
  Constant11/1 -> Mux/12
  Constant10/1 -> Mux/11
  Constant9/1 -> Mux/10
  Constant8/1 -> Mux/9
  Constant7/1 -> Mux/8
  Constant6/1 -> Mux/7
  Constant5/1 -> Mux/6
  Constant4/1 -> Mux/5
  Constant3/1 -> Mux/4
  Constant2/1 -> Mux/3
  Constant1/1 -> Mux/2
  Constant/1 -> Mux/1

== system SIL_OlfatiSaber/UAV 4/Low-level/Autopilot/Altitude Control ==
  Altitude Ref : Inport
  Altitude : Inport  Port=2
  Constant : Constant
  Constant1 : Constant  Value=0.00
  Constant2 : Constant  Value=0.0162
  Constant3 : Constant  Value=10
  Discrete PID : slpidlib/PID Controller  Controller=PID  Form=Parallel  TimeDomain=Discrete-time  UseExternalTs=off  SampleTime=-1  IntegratorMethod=Forward Euler  FilterMethod=Forward Euler  ControllerParametersSource=external  P=1  I=1  D=0  UseFilter=on  N=100  TunerSelectOption=Transfer Function Based (PID Tuner App)  InitialConditionSource=internal  InitialConditionForIntegrator=0  InitialConditionForFilter=0  DifferentiatorICPrevScaledInput=0  ExternalReset=none  TrackingMode=off  Kt=1  LimitOutput=off  SatLimitsSource=internal  UpperSaturationLimit=inf  LowerSaturationLimit=-inf  LinearizeAsGain=on  AntiWindupMode=none  Kb=1  POutMin=[]  POutMax=[]  IOutMin=[]  IOutMax=[]  DOutMin=[]  DOutMax=[]  NOutMin=[]  NOutMax=[]  SumOutMin=[]  SumOutMax=[]  SaturationOutMin=[]  SaturationOutMax=[]  PParamMin=[]  PParamMax=[]  IParamMin=[]  IParamMax=[]  DParamMin=[]  DParamMax=[]  NParamMin=[]  NParamMax=[]  KbParamMin=[]  KbParamMax=[]  KtParamMin=[]  KtParamMax=[]  KbOutMin=[]  KbOutMax=[]  KtOutMin=[]  KtOutMax=[]  IntegratorOutMin=[]  IntegratorOutMax=[]  FilterOutMin=[]  FilterOutMax=[]  SumI1OutMin=[]  SumI1OutMax=[]  SumI2OutMin=[]  SumI2OutMax=[]  SumI3OutMin=[]  SumI3OutMax=[]  SumI4OutMin=[]  SumI4OutMax=[]  SumDOutMin=[]  SumDOutMax=[]  DifferentiatorOutMin=[]  DifferentiatorOutMax=[]  FilterDiffOutCoefMin=[]  FilterDiffOutCoefMax=[]  ReciprocalOutMin=[]  ReciprocalOutMax=[]  SumDenOutMin=[]  SumDenOutMax=[]  SumNumOutMin=[]  SumNumOutMax=[]  DivideOutMin=[]  DivideOutMax=[]  UdiffTsProdOutMin=[]  UdiffTsProdOutMax=[]  NTsProdOutMin=[]  NTsProdOutMax=[]  UintegralTsProdOutMin=[]  UintegralTsProdOutMax=[]  UngainTsProdOutMin=[]  UngainTsProdOutMax=[]  IntegratorContinuousStateAttributes=''  IntegratorStateMustResolveToSignalObject=off  IntegratorRTWStateStorageClass=Auto  FilterContinuousStateAttributes=''  FilterStateMustResolveToSignalObject=off  FilterRTWStateStorageClass=Auto  ParallelPVariant=ExternalParameters  IdealPVariant=Disabled  IVariant=ExternalParameters  DVariant=ExternalParameters  IntegratorVariant=Discrete  SatVariant=Disabled  AWVariant=Passthrough  PCopyVariant=Disabled  TRVariant=Disabled  FdbkBlocksVariant=Forward  IdealPFdbkVariant=Disabled  SatFdbkVariant=Disabled  DerivativeFilterVariant=ForwardEulerFilter  NVariant=ExternalParameters  NCopyVariant=Disabled  FilterICVariant=InternalICsFilter  IntegratorICVariant=InternalICs  ExternalResetVariant=Disabled  TRSumVariant=Passthrough  SumFdbkVariant=Disabled  SumVariant=Sum_PID  TsampFilterVariant=InternalTs  TsampNgainVariant=Passthrough  TsampIntegralVariant=Passthrough  ExternalSaturationOutDataTypeStr=Inherit: Same as second input
  Gain : Gain  Gain=0.1
  Saturation : Saturate  UpperLimit=0.78  LowerLimit=-0.78
  Sum : Sum  Inputs=|+-
  Pitch_ref : Outport
  altitude_error : Outport  Port=2
  wires:
  Saturation/1 -> Pitch_ref/1
  Altitude Ref/1 -> Sum/1
  Altitude/1 -> Sum/2
  Sum/1 -> altitude_error/1, Gain/1
  Constant/1 -> Discrete PID/2
  Constant1/1 -> Discrete PID/3
  Constant2/1 -> Discrete PID/4
  Constant3/1 -> Discrete PID/5
  Discrete PID/1 -> Saturation/1
  Gain/1 -> Discrete PID/1

== system SIL_OlfatiSaber/UAV 4/Low-level/Autopilot/Attitude Control ==
  Pitch Ref : Inport
  Roll_ref : Inport  Port=2
  Euler angles : Inport  Port=3
  Bus Selector1 : BusSelector  OutputSignals=Pitch,Yaw,Roll
  Sum1 : Sum  Inputs=|+-
  Sum3 : Sum  Inputs=+-|
  Terminator : Terminator
  pitch_error : Outport
  roll_error : Outport  Port=2
  wires:
  Euler angles/1 -> Bus Selector1/1
  Sum1/1 -> roll_error/1
  Sum3/1 -> pitch_error/1
  Roll_ref/1 -> Sum1/1
  Bus Selector1/1 -> Sum3/2  "<Pitch>"
  Pitch Ref/1 -> Sum3/1
  Bus Selector1/3 -> Sum1/2  "<Roll>"
  Bus Selector1/2 -> Terminator/1  "<Yaw>"

== system SIL_OlfatiSaber/UAV 4/Low-level/Autopilot/Takeoff ==
  Elevator Command : Inport
  Ailerons Command : Inport  Port=2
  Propeller Command : Inport  Port=3
  Altitude : Inport  Port=4
  Constant1 : Constant  Value=0.0436332
  Constant2 : Constant  Value=0.017
  Constant3 : Constant  Value=0.8
  Constant4 : Constant  Value=0
  Constant5 : Constant  Value=-0.035
  GreaterThanOrEqual : RelationalOperator  OutDataTypeStr=boolean  RndMeth=Simplest
  Switch{1..4} (4 alike) : Switch  Criteria=u2 ~= 0
  altitude takeoff : Constant  Value=5
  profundor : Outport
  aileron : Outport  Port=2
  throtlle : Outport  Port=3
  rudder : Outport  Port=4
  wires:
  Elevator Command/1 -> Switch3/1
  Switch3/1 -> profundor/1
  Ailerons Command/1 -> Switch1/1
  Switch1/1 -> aileron/1
  Switch2/1 -> throtlle/1
  Propeller Command/1 -> Switch2/1
  Constant1/1 -> Switch3/3
  Constant2/1 -> Switch1/3
  Constant3/1 -> Switch2/3
  altitude takeoff/1 -> GreaterThanOrEqual/2
  Altitude/1 -> GreaterThanOrEqual/1
  GreaterThanOrEqual/1 -> Switch4/2, Switch3/2, Switch1/2, Switch2/2
  Constant4/1 -> Switch4/1
  Constant5/1 -> Switch4/3
  Switch4/1 -> rudder/1

== system SIL_OlfatiSaber/UAV 4/Low-level/Autopilot/Velocity Control ==
  Velocity Ref : Inport
  Velocity : Inport  Port=2
  Constant : Constant
  Constant1 : Constant  Value=0.00
  Constant2 : Constant  Value=0.009
  Constant3 : Constant  Value=10
  Discrete PID : slpidlib/PID Controller  Controller=PID  Form=Parallel  TimeDomain=Discrete-time  UseExternalTs=off  SampleTime=-1  IntegratorMethod=Forward Euler  FilterMethod=Forward Euler  ControllerParametersSource=external  P=1  I=1  D=0  UseFilter=on  N=100  TunerSelectOption=Transfer Function Based (PID Tuner App)  InitialConditionSource=internal  InitialConditionForIntegrator=0  InitialConditionForFilter=0  DifferentiatorICPrevScaledInput=0  ExternalReset=none  TrackingMode=off  Kt=1  LimitOutput=off  SatLimitsSource=internal  UpperSaturationLimit=inf  LowerSaturationLimit=-inf  LinearizeAsGain=on  AntiWindupMode=none  Kb=1  POutMin=[]  POutMax=[]  IOutMin=[]  IOutMax=[]  DOutMin=[]  DOutMax=[]  NOutMin=[]  NOutMax=[]  SumOutMin=[]  SumOutMax=[]  SaturationOutMin=[]  SaturationOutMax=[]  PParamMin=[]  PParamMax=[]  IParamMin=[]  IParamMax=[]  DParamMin=[]  DParamMax=[]  NParamMin=[]  NParamMax=[]  KbParamMin=[]  KbParamMax=[]  KtParamMin=[]  KtParamMax=[]  KbOutMin=[]  KbOutMax=[]  KtOutMin=[]  KtOutMax=[]  IntegratorOutMin=[]  IntegratorOutMax=[]  FilterOutMin=[]  FilterOutMax=[]  SumI1OutMin=[]  SumI1OutMax=[]  SumI2OutMin=[]  SumI2OutMax=[]  SumI3OutMin=[]  SumI3OutMax=[]  SumI4OutMin=[]  SumI4OutMax=[]  SumDOutMin=[]  SumDOutMax=[]  DifferentiatorOutMin=[]  DifferentiatorOutMax=[]  FilterDiffOutCoefMin=[]  FilterDiffOutCoefMax=[]  ReciprocalOutMin=[]  ReciprocalOutMax=[]  SumDenOutMin=[]  SumDenOutMax=[]  SumNumOutMin=[]  SumNumOutMax=[]  DivideOutMin=[]  DivideOutMax=[]  UdiffTsProdOutMin=[]  UdiffTsProdOutMax=[]  NTsProdOutMin=[]  NTsProdOutMax=[]  UintegralTsProdOutMin=[]  UintegralTsProdOutMax=[]  UngainTsProdOutMin=[]  UngainTsProdOutMax=[]  IntegratorContinuousStateAttributes=''  IntegratorStateMustResolveToSignalObject=off  IntegratorRTWStateStorageClass=Auto  FilterContinuousStateAttributes=''  FilterStateMustResolveToSignalObject=off  FilterRTWStateStorageClass=Auto  ParallelPVariant=ExternalParameters  IdealPVariant=Disabled  IVariant=ExternalParameters  DVariant=ExternalParameters  IntegratorVariant=Discrete  SatVariant=Disabled  AWVariant=Passthrough  PCopyVariant=Disabled  TRVariant=Disabled  FdbkBlocksVariant=Forward  IdealPFdbkVariant=Disabled  SatFdbkVariant=Disabled  DerivativeFilterVariant=ForwardEulerFilter  NVariant=ExternalParameters  NCopyVariant=Disabled  FilterICVariant=InternalICsFilter  IntegratorICVariant=InternalICs  ExternalResetVariant=Disabled  TRSumVariant=Passthrough  SumFdbkVariant=Disabled  SumVariant=Sum_PID  TsampFilterVariant=InternalTs  TsampNgainVariant=Passthrough  TsampIntegralVariant=Passthrough  ExternalSaturationOutDataTypeStr=Inherit: Same as second input
  K_prop : Gain  Gain=0.1
  Sum1 : Sum  Inputs=|++
  Sum7 : Sum  Inputs=|+-
  propeller_ref : Constant  Value=0.64
  propeller_cmd : Outport
  velocity_error : Outport  Port=2
  wires:
  Velocity/1 -> Sum7/2
  Velocity Ref/1 -> Sum7/1
  Sum7/1 -> velocity_error/1, K_prop/1
  Sum1/1 -> propeller_cmd/1
  propeller_ref/1 -> Sum1/2
  Constant3/1 -> Discrete PID/5
  Constant/1 -> Discrete PID/2
  Discrete PID/1 -> Sum1/1
  Constant1/1 -> Discrete PID/3
  K_prop/1 -> Discrete PID/1
  Constant2/1 -> Discrete PID/4
